simulink model "MeasurementSystem"  (R2020a)
settings: Solver=VariableStepAuto  StartTime=0.0  StopTime=10.0  RelTol=1e-3
undefined symbols (not defined in the file): P, Ts
libraries: simulink x10, powerlib_meascontrol x1
settings Model: Creator=Sony  LastModifiedBy=Sony

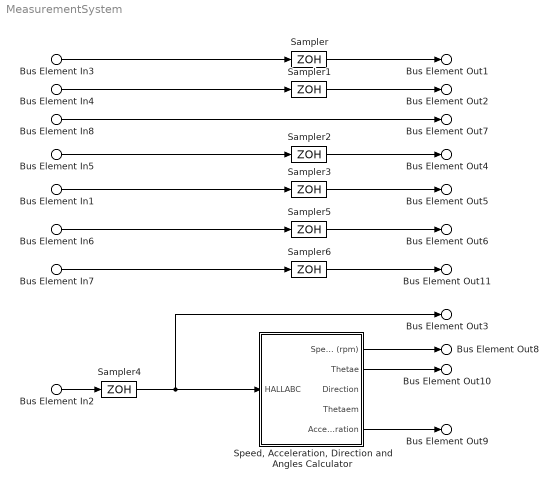
== system MeasurementSystem ==
  Bus Element In3 : Inport  PortName=DC Voltage VDC
  Bus Element In4 : Inport  Port=2  PortName=DC Current IDC
  Bus Element In5 : Inport  Port=3  PortName=AC Stator Voltages VABC
  Bus Element In1 : Inport  Port=4  PortName=AC Stator Currents IABC
  Bus Element In2 : Inport  Port=5  PortName=HALL Sensor Signals HABC
  Bus Element In6 : Inport  Port=6  PortName=Temperature
  Bus Element In7 : Inport  Port=7  PortName=Reference Speed (rpm)
  Bus Element In8 : Inport  Port=8  PortName=Inverter Gatings
  Sampler{,1..6} (7 alike) : ZeroOrderHold  SampleTime=1e-4
  "Speed, Acceleration, Direction and Angles Calculator" : Subsystem
  Bus Element Out1 : Outport  PortName=Sampled DC Input Voltage VDC
  Bus Element Out2 : Outport  Port=2  PortName=Sampled DC Input Current IDC
  Bus Element Out4 : Outport  Port=3  PortName=Sampled Stator VABC
  Bus Element Out5 : Outport  Port=4  PortName=Sampled Stator IABC
  Bus Element Out3 : Outport  Port=5  PortName=Sampled HALL Signals HABC
  Bus Element Out6 : Outport  Port=6  PortName=Sampled Temperature
  Bus Element Out8 : Outport  Port=7  PortName=Sampled Speed (rpm)
  Bus Element Out7 : Outport  Port=8  PortName=Sampled Inverter Gatings
  Bus Element Out9 : Outport  Port=9  PortName=Sampled Acceleration
  Bus Element Out10 : Outport  Port=10  PortName=Sampled Rotor Electrical Angle
  Bus Element Out11 : Outport  Port=11  PortName=Sampled Reference Speed (rpm)
  wires:
  Sampler3/1 -> Bus Element Out5/1
  Bus Element In1/1 -> Sampler3/1
  "Speed, Acceleration, Direction and Angles Calculator"/1(Speed (rpm)) -> Bus Element Out8/1
  Bus Element In6/1 -> Sampler5/1
  Bus Element In8/1 -> Bus Element Out7/1
  Bus Element In7/1 -> Sampler6/1
  Sampler1/1 -> Bus Element Out2/1
  Sampler4/1 -> Bus Element Out3/1, "Speed, Acceleration, Direction and Angles Calculator"/1(HALLABC)
  Bus Element In2/1 -> Sampler4/1
  Sampler2/1 -> Bus Element Out4/1
  Bus Element In4/1 -> Sampler1/1
  Bus Element In3/1 -> Sampler/1
  Sampler6/1 -> Bus Element Out11/1
  "Speed, Acceleration, Direction and Angles Calculator"/5(Acceleration) -> Bus Element Out9/1
  "Speed, Acceleration, Direction and Angles Calculator"/2(Thetae) -> Bus Element Out10/1
  Sampler5/1 -> Bus Element Out6/1
  Sampler/1 -> Bus Element Out1/1
  Bus Element In5/1 -> Sampler2/1

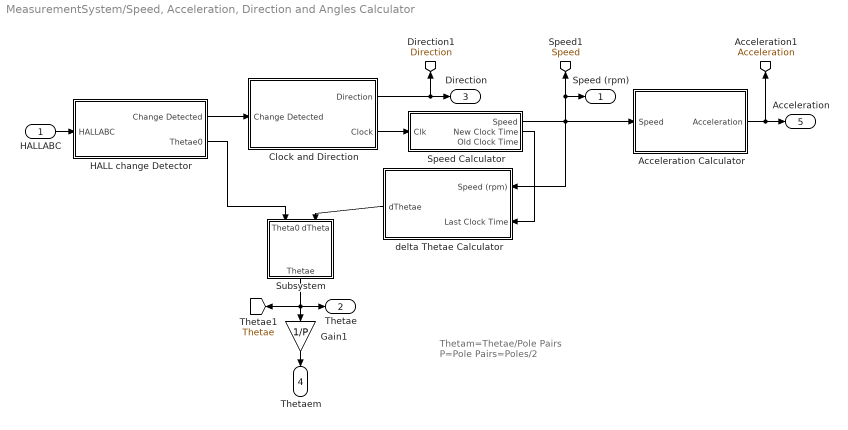
== system MeasurementSystem/Speed, Acceleration, Direction and Angles Calculator ==
  note: Thetam=Thetae/Pole Pairs
      | P=Pole Pairs=Poles/2
  HALLABC : Inport
  Acceleration Calculator : Subsystem
  Clock and Direction : Subsystem
  Gain1 : Gain  Gain=1/P
  HALL change Detector : Subsystem
  Speed Calculator : Subsystem
  Subsystem : Subsystem
  delta Thetae Calculator : Subsystem
  Speed (rpm) : Outport
  Thetae : Outport  Port=2
  Direction : Outport  Port=3
  Thetaem : Outport  Port=4
  Acceleration : Outport  Port=5
  tag scope: Acceleration=global, Direction=global, Speed=global, Thetae=global
  wires:
  HALLABC/1 -> HALL change Detector/1(HALLABC)
  Clock and Direction/2(Clock) -> Speed Calculator/1(Clk)
  HALL change Detector/1(Change Detected) -> Clock and Direction/1(Change Detected)
  Clock and Direction/1(Direction) -> Direction/1, [Direction]
  Speed Calculator/2(New Clock Time) -> delta Thetae Calculator/2(Last Clock Time)
  Acceleration Calculator/1(Acceleration) -> [Acceleration], Acceleration/1
  Speed Calculator/1(Speed) -> delta Thetae Calculator/1(Speed (rpm)), Acceleration Calculator/1(Speed), Speed (rpm)/1, [Speed]
  HALL change Detector/2(Thetae0) -> Subsystem/1(Theta0)
  delta Thetae Calculator/1(dThetae) -> Subsystem/2(dTheta)
  Gain1/1 -> Thetaem/1
  Subsystem/1(Thetae) -> Thetae/1, Gain1/1, [Thetae]

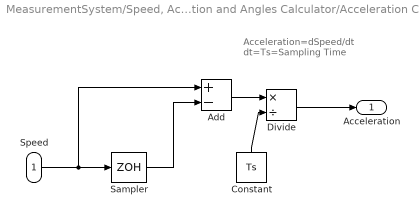
== system MeasurementSystem/Speed, Acceleration, Direction and Angles Calculator/Acceleration Calculator ==
  note: Acceleration=dSpeed/dt
      | dt=Ts=Sampling Time
  Speed : Inport
  Add : Sum  Inputs=+-
  Constant : Constant  Value=Ts
  Divide : Product  Inputs=*/
  Sampler : ZeroOrderHold  SampleTime=Ts
  Acceleration : Outport
  wires:
  Speed/1 -> Add/1, Sampler/1
  Sampler/1 -> Add/2
  Add/1 -> Divide/1
  Constant/1 -> Divide/2
  Divide/1 -> Acceleration/1

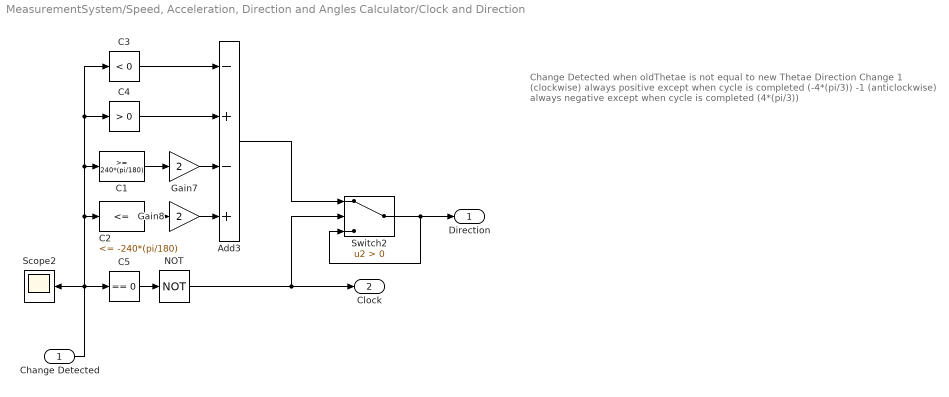
== system MeasurementSystem/Speed, Acceleration, Direction and Angles Calculator/Clock and Direction ==
  note: Change Detected when oldThetae
      | is not equal to new Thetae
      |
      | Direction                                                                                               Change
      | 1 (clockwise)                       always positive except when cycle is completed (-4*(pi/3))
      | -1 (anticlockwise)                 always negative except when cycle is completed (4*(pi/3))
  Change Detected : Inport
  Add3 : Sum  Inputs=-+-+  OutDataTypeStr=double
  C1 : simulink/Logic and Bit Operations/Compare To Constant  relop=>=  const=240*(pi/180)  OutDataTypeStr=boolean
  C2 : simulink/Logic and Bit Operations/Compare To Constant  relop=<=  const=-240*(pi/180)  OutDataTypeStr=boolean
  C3 : simulink/Logic and Bit Operations/Compare To Zero  relop=<  OutDataTypeStr=boolean
  C4 : simulink/Logic and Bit Operations/Compare To Zero  relop=>  OutDataTypeStr=boolean
  C5 : simulink/Logic and Bit Operations/Compare To Zero  relop===  OutDataTypeStr=boolean
  Gain7 : Gain  Gain=2
  Gain8 : Gain  Gain=2
  NOT : Logic  Operator=NOT  AllPortsSameDT=off  OutDataTypeStr=boolean
  Scope2 : Scope
  Switch2 : Switch  Criteria=u2 > Threshold
  Direction : Outport
  Clock : Outport  Port=2
  wires:
  Change Detected/1 -> Scope2/1, C5/1, C2/1, C1/1, C4/1, C3/1
  C3/1 -> Add3/1
  C5/1 -> NOT/1
  Add3/1 -> Switch2/1
  Gain7/1 -> Add3/3
  Gain8/1 -> Add3/4
  NOT/1 -> Switch2/2, Clock/1
  C4/1 -> Add3/2
  C1/1 -> Gain7/1
  C2/1 -> Gain8/1
  Switch2/1 -> Switch2/3, Direction/1

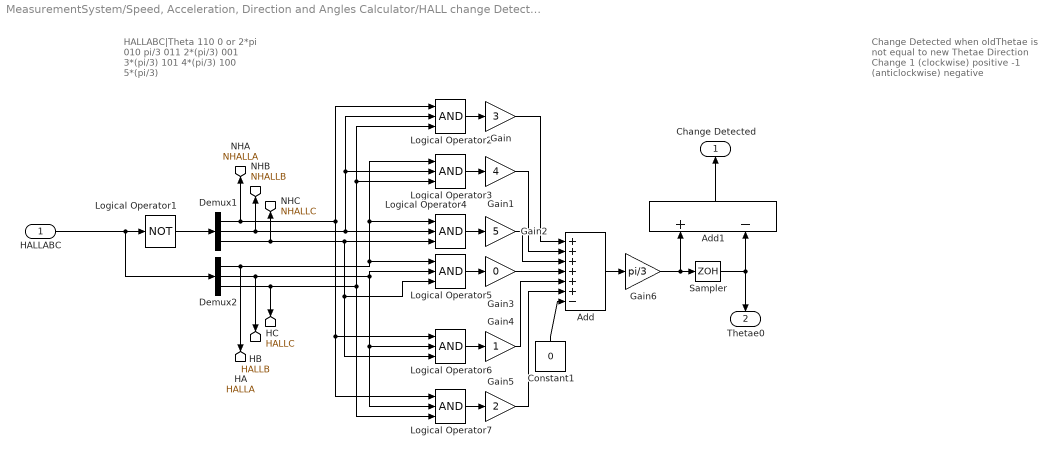
== system MeasurementSystem/Speed, Acceleration, Direction and Angles Calculator/HALL change Detector ==
  note: Change Detected when oldThetae
      | is not equal to new Thetae
      |
      | Direction                         Change
      | 1 (clockwise)                        positive
      | -1 (anticlockwise)                 negative
  note: HALLABC|Theta
      | 110    0 or 2*pi
      | 010           pi/3
      | 011     2*(pi/3)
      | 001      3*(pi/3)
      | 101      4*(pi/3)
      | 100     5*(pi/3)
  HALLABC : Inport
  Add : Sum  Inputs=++++++-
  Add1 : Sum  Inputs=+-
  Constant1 : Constant  Value=0
  Demux1 : Demux  Outputs=3
  Demux2 : Demux  Outputs=3
  Gain : Gain  Gain=3
  Gain1 : Gain  Gain=4
  Gain2 : Gain  Gain=5
  Gain3 : Gain  Gain=0
  Gain4 : Gain
  Gain5 : Gain  Gain=2
  Gain6 : Gain  Gain=pi/3  ParamDataTypeStr=double
  Logical Operator1 : Logic  Operator=NOT  AllPortsSameDT=off  OutDataTypeStr=boolean
  Logical Operator{2..7} (6 alike) : Logic  Inputs=3  AllPortsSameDT=off  OutDataTypeStr=boolean
  Sampler : ZeroOrderHold  SampleTime=1.01*Ts
  Change Detected : Outport
  Thetae0 : Outport  Port=2
  tag scope: HALLA=global, HALLB=global, HALLC=global, NHALLA=global, NHALLB=global, NHALLC=global
  wires:
  Logical Operator6/1 -> Gain4/1
  Gain/1 -> Add/1
  Logical Operator3/1 -> Gain1/1
  Gain1/1 -> Add/2
  Add1/1 -> Change Detected/1
  Add/1 -> Gain6/1
  Demux1/1 -> [NHALLA], Logical Operator7/1, Logical Operator6/1, Logical Operator2/1
  Gain2/1 -> Add/3
  Demux2/3 -> Logical Operator7/3, Logical Operator3/3, Logical Operator2/3, [HALLC]
  Demux2/1 -> [HALLA], Logical Operator4/1, Logical Operator3/1, Logical Operator5/1
  Logical Operator1/1 -> Demux1/1
  Logical Operator5/1 -> Gain3/1
  Demux1/2 -> Logical Operator3/2, Logical Operator2/2, Logical Operator4/2, [NHALLB]
  Demux2/2 -> Logical Operator6/2, Logical Operator7/2, Logical Operator5/2, [HALLB]
  Gain4/1 -> Add/5
  Logical Operator4/1 -> Gain2/1
  HALLABC/1 -> Logical Operator1/1, Demux2/1
  Gain6/1 -> Add1/1, Sampler/1
  Gain5/1 -> Add/6
  Logical Operator7/1 -> Gain5/1
  Logical Operator2/1 -> Gain/1
  Gain3/1 -> Add/4
  Demux1/3 -> Logical Operator6/3, Logical Operator5/3, Logical Operator4/3, [NHALLC]
  Sampler/1 -> Thetae0/1, Add1/2
  Constant1/1 -> Add/7

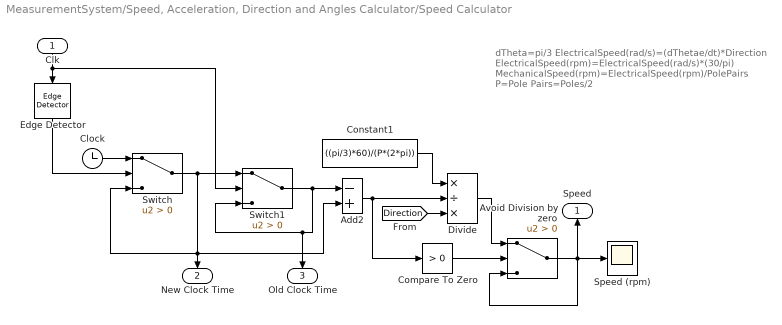
== system MeasurementSystem/Speed, Acceleration, Direction and Angles Calculator/Speed Calculator ==
  note: dTheta=pi/3
      | ElectricalSpeed(rad/s)=(dThetae/dt)*Direction
      | ElectricalSpeed(rpm)=ElectricalSpeed(rad/s)*(30/pi)
      | MechanicalSpeed(rpm)=ElectricalSpeed(rpm)/PolePairs
      | P=Pole Pairs=Poles/2
  Clk : Inport
  Add2 : Sum  Inputs=-+
  Avoid Division by zero : Switch  Criteria=u2 > Threshold
  Clock : Clock
      settings: Decimation=1000000
  Compare To Zero : simulink/Logic and Bit Operations/Compare To Zero  relop=>  OutDataTypeStr=boolean
  Constant1 : Constant  Value=((pi/3)*60)/(P*(2*pi))
  Divide : Product  Inputs=*/*  LockScale=on
  Edge Detector : powerlib_meascontrol/Logic/Edge Detector  model=Falling  ic=0  Ts=-1
      settings: SourceProductBaseCode=PS
  Speed (rpm) : Scope
  Switch : Switch  Criteria=u2 > Threshold
  Switch1 : Switch  Criteria=u2 > Threshold
  Speed : Outport
  New Clock Time : Outport  Port=2
  Old Clock Time : Outport  Port=3
  wires:
  Clk/1 -> Edge Detector/1, Switch1/2
  Divide/1 -> Avoid Division by zero/1
  Constant1/1 -> Divide/1
  Clock/1 -> Switch/1
  Switch1/1 -> Old Clock Time/1, Switch1/3, Add2/1
  [Direction] -> Divide/3
  Add2/1 -> Compare To Zero/1, Divide/2
  Edge Detector/1 -> Switch/2
  Switch/1 -> Add2/2, New Clock Time/1, Switch/3, Switch1/1
  Compare To Zero/1 -> Avoid Division by zero/2
  Avoid Division by zero/1 -> Speed/1, Speed (rpm)/1, Avoid Division by zero/3

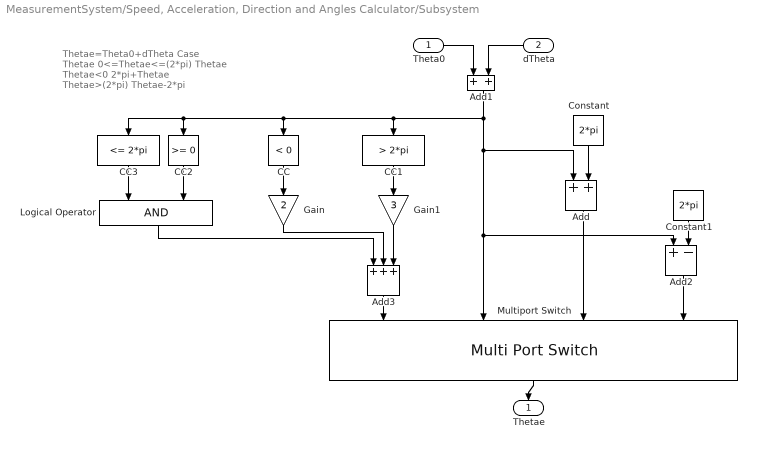
== system MeasurementSystem/Speed, Acceleration, Direction and Angles Calculator/Subsystem ==
  note: Thetae=Theta0+dTheta
      | Case                                 Thetae
      | 0<=Thetae<=(2*pi)           Thetae
      | Thetae<0                 2*pi+Thetae
      | Thetae>(2*pi)           Thetae-2*pi
  Theta0 : Inport
  dTheta : Inport  Port=2
  Add : Sum
  Add1 : Sum
  Add2 : Sum  Inputs=+-
  Add3 : Sum  Inputs=+++
  CC : simulink/Logic and Bit Operations/Compare To Constant  relop=<  const=0  OutDataTypeStr=boolean
  CC1 : simulink/Logic and Bit Operations/Compare To Constant  relop=>  const=2*pi  OutDataTypeStr=boolean
  CC2 : simulink/Logic and Bit Operations/Compare To Constant  relop=>=  const=0  OutDataTypeStr=boolean
  CC3 : simulink/Logic and Bit Operations/Compare To Constant  relop=<=  const=2*pi  OutDataTypeStr=boolean
  Constant : Constant  Value=2*pi
  Constant1 : Constant  Value=2*pi
  Gain : Gain  Gain=2
  Gain1 : Gain  Gain=3
  Logical Operator : Logic  AllPortsSameDT=off  OutDataTypeStr=boolean
  Multiport Switch : MultiPortSwitch
  Thetae : Outport
  wires:
  Theta0/1 -> Add1/1
  dTheta/1 -> Add1/2
  Constant1/1 -> Add2/2
  Constant/1 -> Add/2
  Add2/1 -> Multiport Switch/4
  Multiport Switch/1 -> Thetae/1
  Add/1 -> Multiport Switch/3
  CC/1 -> Gain/1
  CC1/1 -> Gain1/1
  CC3/1 -> Logical Operator/1
  CC2/1 -> Logical Operator/2
  Add3/1 -> Multiport Switch/1
  Gain1/1 -> Add3/3
  Gain/1 -> Add3/2
  Logical Operator/1 -> Add3/1
  Add1/1 -> CC2/1, CC3/1, CC/1, CC1/1, Add2/1, Multiport Switch/2, Add/1

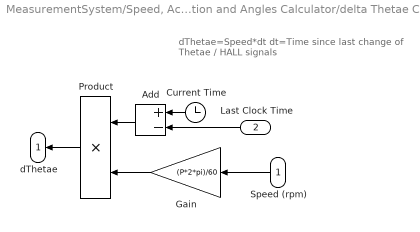
== system MeasurementSystem/Speed, Acceleration, Direction and Angles Calculator/delta Thetae Calculator ==
  note: dThetae=Speed*dt
      | dt=Time since last change of Thetae / HALL signals
  Speed (rpm) : Inport
  Last Clock Time : Inport  Port=2
  Add : Sum  Inputs=+-
  Current Time : Clock
      settings: Decimation=1000000
  Gain : Gain  Gain=(P*2*pi)/60
  Product : Product
  dThetae : Outport
  wires:
  Last Clock Time/1 -> Add/2
  Current Time/1 -> Add/1
  Gain/1 -> Product/2
  Product/1 -> dThetae/1
  Add/1 -> Product/1
  Speed (rpm)/1 -> Gain/1
